simulink model "signalgeneration_rev2"  (Simulink 7.5)
settings: Solver=ode1  StartTime=0.0  StopTime=100  FixedStep=0.01  RelTol=1e-3
libraries: simulink x1
settings Model: Creator=s13071832  LastModifiedBy=s13071832

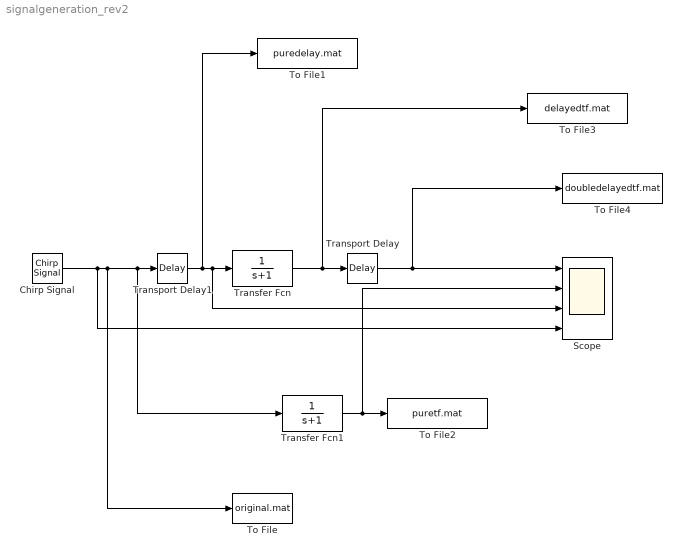
== system signalgeneration_rev2 ==
  Chirp Signal : simulink/Sources/Chirp Signal  SystemSampleTime=-1  f1=0.1  T=100  f2=1
  Scope : Scope  NumInputPorts=4
      settings: YMin=-5~-5~-5~-5  YMax=5~5~5~5
  To File : ToFile  Filename=original.mat  SaveFormat=Timeseries
  To File1 : ToFile  Filename=puredelay.mat  SaveFormat=Timeseries
  To File2 : ToFile  Filename=puretf.mat  SaveFormat=Timeseries
  To File3 : ToFile  Filename=delayedtf.mat  SaveFormat=Timeseries
  To File4 : ToFile  Filename=doubledelayedtf.mat  SaveFormat=Timeseries
  Transfer Fcn : TransferFcn  Denominator=[1 1]
  Transfer Fcn1 : TransferFcn  Denominator=[1 1]
  Transport Delay : TransportDelay  DelayTime=3
  Transport Delay1 : TransportDelay  DelayTime=6.3
  wires:
  Transfer Fcn/1 -> Transport Delay/1, To File3/1
  Transport Delay/1 -> To File4/1, Scope/1
  Transport Delay1/1 -> To File1/1, Transfer Fcn/1, Scope/3
  Transfer Fcn1/1 -> To File2/1, Scope/2
  Chirp Signal/1 -> To File/1, Transport Delay1/1, Transfer Fcn1/1, Scope/4
